simulink model "instrumentation_amplifier"  (R2025b)
settings: Solver=ode23t  StartTime=0.0  StopTime=10  RelTol=1e-4  EnableMultiTasking=on
libraries: fl_lib x14, dspfdesign x3, nesl_utility x3
settings Model: PacingRate=0.100000  Creator=lenovo  LastModifiedBy=saif
settings SolverCC: AlgebraicLoopSolver=TrustRegion
settings DataIOCC: LimitDataPoints=on  SaveFormat=Array  SignalLoggingSaveFormat=ModelDataLogs  ReturnWorkspaceOutputs=off
settings OptimizationCC: ExpressionDepthLimit=2147483647.0  LifeSpan=inf
settings DebuggingCC: UnderspecifiedInitializationDetection=Classic  MergeDetectMultiDrivingBlocksExec=none  SolverPrmCheckMsg=warning  FcnCallInpInsideContextMsg=warning  UnconnectedInputMsg=warning  UnconnectedOutputMsg=warning  UnconnectedLineMsg=warning  StateNameClashWarn=warning  SFUnexpectedBacktrackingDiag=warning  SFNoUnconditionalDefaultTransitionDiag=warning  SFExecutionAtInitializationDiag=none  ArithmeticOperatorsInVariantConditions=warning
settings HardwareCC: ProdBitPerPointer=32.0  ProdBitPerSizeT=32.0  ProdBitPerPtrDiffT=32.0  ProdLargestAtomicFloat=None  ProdIntDivRoundTo=Undefined  ProdEndianess=Unspecified  ProdWordSize=32.0  ProdHWDeviceType=32-bit Generic
settings ModelReferenceCC: PropagateSignalLabelsOutOfModel=off
settings SFSimCC: SimUseLocalCustomCode=off  CustomCodeUndefinedFunction=UseInterfaceOnly
settings RTWCC: RTWUseLocalCustomCode=off  GPUComputeCapability=3.5
settings CodeAppCC: StateflowObjectComments=on
settings GRTTargetCC: TargetLangStandard=C89/C90 (ANSI)  CombineOutputUpdateFcns=off  GRTInterface=on
settings ConfigComp: CovMetricSettings=dw  CovSaveCumulativeToWorkspaceVar=on  CovSaveSingleToWorkspaceVar=on  CovExternalEMLEnable=off
settings SimscapeCC: ExplicitSolverDiagnosticOptions=none  SimscapeNormalizeSystem=off

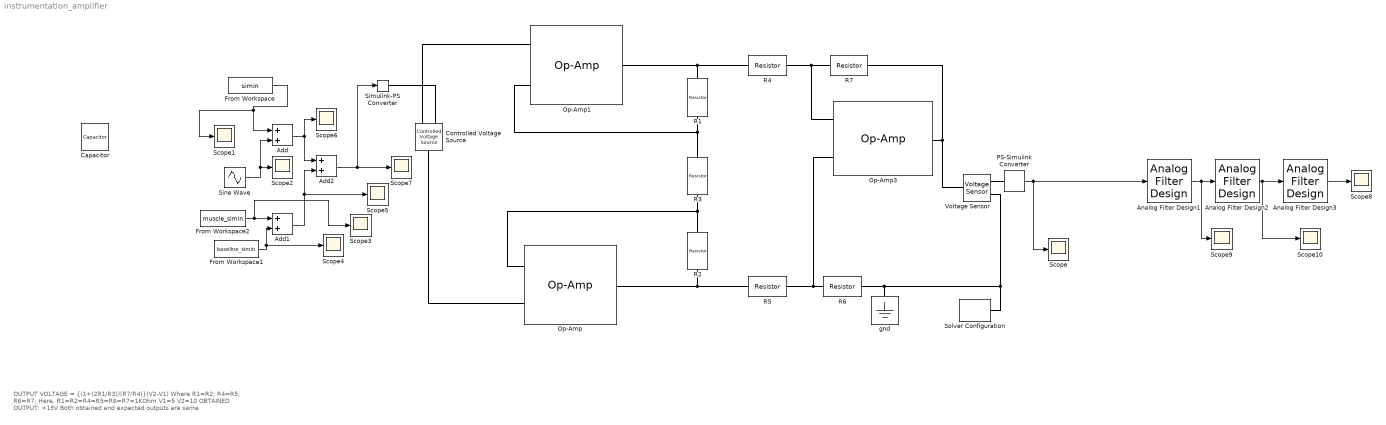
== system instrumentation_amplifier ==
  note: OUTPUT VOLTAGE =  {(1+(2R1/R3))(R7/R4)}(V2-V1)
      | Where
      | R1=R2;
      | R4=R5;
      | R6=R7;
      |
      | Here,
      | R1=R2=R4=R5=R6=R7=1KOhm
      | V1=5
      | V2=10
      |
      | OBTAINED OUTPUT:  +15V
      |
      | Both obtained and expected outputs are same
  Add : Sum
  Add1 : Sum
  Add2 : Sum
  Analog Filter Design1 : dspfdesign/Analog Filter Design  method=Chebyshev II  filttype=Highpass  N=6  Wlo=2*pi*0.5  Whi=80  Rp=2  Rs=80
  Analog Filter Design2 : dspfdesign/Analog Filter Design  method=Chebyshev II  filttype=Lowpass  N=12  Wlo=35*pi*2  Whi=80  Rp=2  Rs=80
  Analog Filter Design3 : dspfdesign/Analog Filter Design  method=Chebyshev II  filttype=Bandstop  N=6  Wlo=2*pi*49  Whi=2*pi*51  Rp=2  Rs=80
  Capacitor : fl_lib/Electrical/Electrical Elements/Capacitor  c=1e-6 F  r=1e-6 Ohm  g=0 1/Ohm  i_specify=off  i_priority=None  i=0 A  i_nominal_specify=off  i_nominal_value=1  i_nominal_unit=A  v_specify=off  v_priority=None  v=0 V  v_nominal_specify=off  v_nominal_value=1  v_nominal_unit=V  vc_specify=on  vc_priority=High  vc=0 V  vc_nominal_specify=off  vc_nominal_value=1  vc_nominal_unit=V
  Controlled Voltage Source : fl_lib/Electrical/Electrical Sources/Controlled Voltage Source
  From Workspace : FromWorkspace  VariableName=simin
  From Workspace1 : FromWorkspace  VariableName=baseline_simin
  From Workspace2 : FromWorkspace  VariableName=muscle_simin
  Op-Amp : fl_lib/Electrical/Electrical Elements/Op-Amp  outI_specify=off  outI_priority=None  outI=0 A  outI_nominal_specify=off  outI_nominal_value=1  outI_nominal_unit=A
  Op-Amp1 : fl_lib/Electrical/Electrical Elements/Op-Amp  outI_specify=off  outI_priority=None  outI=0 A  outI_nominal_specify=off  outI_nominal_value=1  outI_nominal_unit=A
  Op-Amp3 : fl_lib/Electrical/Electrical Elements/Op-Amp  outI_specify=off  outI_priority=None  outI=0 A  outI_nominal_specify=off  outI_nominal_value=1  outI_nominal_unit=A
  PS-Simulink Converter : nesl_utility/PS-Simulink Converter  PhysicalDomain=network_engine_domain  SubClassName=ps_output  LeftPortType=input  RightPortType=output  PseudoPeriodic=off  Frequencies=[]  VectorFormat=1-D array  Unit=1  AffineConversion=off
  R1 : fl_lib/Electrical/Electrical Elements/Resistor  R=4500 Ohm  i_specify=off  i_priority=None  i=0 A  i_nominal_specify=off  i_nominal_value=1  i_nominal_unit=A  v_specify=off  v_priority=None  v=0 V  v_nominal_specify=off  v_nominal_value=1  v_nominal_unit=V
  R2 : fl_lib/Electrical/Electrical Elements/Resistor  R=4500 Ohm  i_specify=off  i_priority=None  i=0 A  i_nominal_specify=off  i_nominal_value=1  i_nominal_unit=A  v_specify=off  v_priority=None  v=0 V  v_nominal_specify=off  v_nominal_value=1  v_nominal_unit=V
  R3 : fl_lib/Electrical/Electrical Elements/Resistor  R=10000 Ohm  i_specify=off  i_priority=None  i=0 A  i_nominal_specify=off  i_nominal_value=1  i_nominal_unit=A  v_specify=off  v_priority=None  v=0 V  v_nominal_specify=off  v_nominal_value=1  v_nominal_unit=V
  R{4..7} (4 alike) : fl_lib/Electrical/Electrical Elements/Resistor  R=1000 Ohm  i_specify=off  i_priority=None  i=0 A  i_nominal_specify=off  i_nominal_value=1  i_nominal_unit=A  v_specify=off  v_priority=None  v=0 V  v_nominal_specify=off  v_nominal_value=1  v_nominal_unit=V
  Scope{,1..10} (11 alike) : Scope
      Scope settings: ActiveDisplayYMinimum=-6.2404200556820433  ActiveDisplayYMaximum=6.190637752385526
      Scope1 settings: ActiveDisplayYMinimum=-0.70980429507339715  ActiveDisplayYMaximum=1.0775338598586357
      Scope10 settings: ActiveDisplayYMinimum=-0.70518941159389281  ActiveDisplayYMaximum=2.7573848449496126  DataLoggingVariableName=ScopeData10
      Scope2 settings: ActiveDisplayYMinimum=-0.4398542620505177  ActiveDisplayYMaximum=0.52871761149995722  DataLoggingVariableName=ScopeData2
      Scope3 settings: ActiveDisplayYMinimum=-1.3775948547515195  ActiveDisplayYMaximum=4.3498360939187357  DataLoggingVariableName=ScopeData3
      Scope4 settings: ActiveDisplayYMinimum=-1.3775948547515195  ActiveDisplayYMaximum=4.3498360939187357  DataLoggingVariableName=ScopeData4
      Scope5 settings: ActiveDisplayYMinimum=-2.3464573354161775  ActiveDisplayYMaximum=0.8843226529527044  DataLoggingVariableName=ScopeData5
      Scope6 settings: ActiveDisplayYMinimum=-0.39095483895706873  ActiveDisplayYMaximum=2.6464240774694021  DataLoggingVariableName=ScopeData6
      Scope7 settings: ActiveDisplayYMinimum=-1.3775948547515195  ActiveDisplayYMaximum=4.3498360939187357  DataLoggingVariableName=ScopeData7
      Scope8 settings: ActiveDisplayYMinimum=-2.1564611923106645  ActiveDisplayYMaximum=1.701169669565024  DataLoggingVariableName=ScopeData8
      Scope9 settings: ActiveDisplayYMinimum=-0.050889623927884542  ActiveDisplayYMaximum=1.4846961092473916  DataLoggingVariableName=ScopeData9
  Simulink-PS Converter : nesl_utility/Simulink-PS Converter  PhysicalDomain=network_engine_domain  SubClassName=ps_input  LeftPortType=input  RightPortType=output  PseudoPeriodic=off  Frequencies=[]  NoiseDistribution=none  NoiseParameters=[]  Unit=1  AffineConversion=off  FilteringAndDerivatives=filter  SimscapeFilterOrder=1  InputFilterTimeConstant=0.001  UdotUserProvided=0
  Sine Wave : Sin  Amplitude=0.2  Frequency=2*pi*50  SampleTime=0.001
  Solver Configuration : nesl_utility/Solver Configuration  PhysicalDomain=network_engine_domain  SubClassName=solver  LeftPortType=input  RightPortType=generic  Tones=[]  Harmonics=[]  SimulateNoise=off  Profile=off  UseLocalSampling=off  EnableSwitchedLinearOptims=on  FrequencyDomain=off  UseCCode=off  RelTol=0.001  AbsTol=0.001  MinStep=1e-09  ToWorkspace=off  RevertToSquareIcSolve=off  NumHomotopyIterations=100  PhasorMode=off  PhasorModeNumHarmonics=1  ConsistencySolver=NEWTON_FTOL  IndexReductionMethod=DerivativeReplacement  DoDC=off  ResidualTolerance=1e-9  ConsistencyTolSource=GLOBAL  ConsistencyAbsTol=0.001  ConsistencyRelTol=0.001  ConsistencyTolFactor=0.001  UseLocalSolver=off  LocalSolverChoice=NE_BACKWARD_EULER_ADVANCER  ResolveIndetEquations=on  FunctionEvalNumThread=1  LocalSolverSampleTime=0.001  DoFixedCost=off  MaxNonlinIter=12  MaxModeIter=2  ComputeImpulses=off  ImpulseIterations=2  LinearAlgebra=Sparse  LinearAlgebraNumThread=0  EquationFormulation=NE_TIME_EF  DelaysMemoryBudget=1024  AutomaticFiltering=on  FilteringTimeConstant=0.001  PartitionStorageMethod=AS_NEEDED  PartitionMemoryBudget=1024  PartitionMethod=FAST  MultibodyUseLocalSolver=off  MultibodyLocalSolverChoice=ODE1  MultibodyLocalSolverSampleTime=0.001
  Voltage Sensor : fl_lib/Electrical/Electrical Sensors/Voltage Sensor
  gnd : fl_lib/Electrical/Electrical Elements/Electrical Reference
  wires:
  From Workspace/1 -> Scope1/1, Add/1
  Sine Wave/1 -> Add/2, Scope2/1
  From Workspace2/1 -> Scope3/1, Add1/1
  From Workspace1/1 -> Scope4/1, Add1/2
  Add2/1 -> Scope7/1, Simulink-PS Converter/1
  Add/1 -> Add2/1, Scope6/1
  Add1/1 -> Add2/2, Scope5/1
  PS-Simulink Converter/1 -> Analog Filter Design1/1, Scope/1
  Analog Filter Design1/1 -> Analog Filter Design2/1, Scope9/1
  Analog Filter Design2/1 -> Scope10/1, Analog Filter Design3/1
  Analog Filter Design3/1 -> Scope8/1
  connections:
  Op-Amp/RConn1 -- R2/RConn1 -- R5/LConn1
  R3/RConn1 -- R2/LConn1 -- Op-Amp/LConn2
  R1/RConn1 -- R3/LConn1 -- Op-Amp1/LConn2
  R1/LConn1 -- Op-Amp1/RConn1 -- R4/LConn1
  R4/RConn1 -- Op-Amp3/LConn2 -- R7/LConn1
  R5/RConn1 -- Op-Amp3/LConn1 -- R6/LConn1
  Solver Configuration/RConn1 -- Voltage Sensor/RConn2 -- R6/RConn1 -- gnd/LConn1
  Op-Amp3/RConn1 -- Voltage Sensor/LConn1 -- R7/RConn1
  Simulink-PS Converter/RConn1 -- Controlled Voltage Source/RConn1
  Controlled Voltage Source/LConn1 -- Op-Amp/LConn1
  Controlled Voltage Source/RConn2 -- Op-Amp1/LConn1
  PS-Simulink Converter/LConn1 -- Voltage Sensor/RConn1
